simulink model "model_without_loop"  (R2022a)
settings: Solver=VariableStepAuto  StartTime=0.0  StopTime=1000  MaxStep=1e-3  RelTol=1e-3
values from neighbouring files (symbols this model uses):
  b_m = b_0    (= 7)    [config.m]
  en1 = zeros(length(Lambda), 1)    [config.m]
  gamma = 10000    [config.m]    (also in task_kras.m = 10000000000; tasks.m = 100000000; test_grad.m = 1000)
  k_0 = 1    [config.m]
  K_M = K_M_g    [config.m]
  Lambda = -k_0    (= -1)    [config.m]
  nu1 = zeros(length(Lambda), 1)    [config.m]
  nu2 = zeros(length(Lambda), 1)    [config.m]
  object_denum = [1 a_1 a_0]    [config.m]
  object_num = [b_0]    [config.m]
  psi_hat_init_conds = zeros(omega_size, 1)    [config.m]
  SysKM = ss(K_M_mat)    [config.m]
  SysMat = ss(Lmat)    [config.m]    (also in test_conf.m)
  SysVec = ss(Lvec)    [config.m]    (also in test_conf.m)
settings Model: SimulationMode=accelerator  LastModifiedBy=Vvlad
settings OptimizationCC: BlockReduction=off  BooleanDataType=off
settings DebuggingCC: SaveWithParameterizedLinksMsg=none  UnderspecifiedInitializationDetection=Classic  MergeDetectMultiDrivingBlocksExec=none  SignalResolutionControl=TryResolveAllWithWarning  UnconnectedInputMsg=warning  UnconnectedOutputMsg=warning  UnconnectedLineMsg=warning  UnderSpecifiedDimensionMsg=warning
settings HardwareCC: TargetUnknown=on
settings ModelReferenceCC: PropagateSignalLabelsOutOfModel=off
settings RTWCC: DLArmComputeVersion=19.05

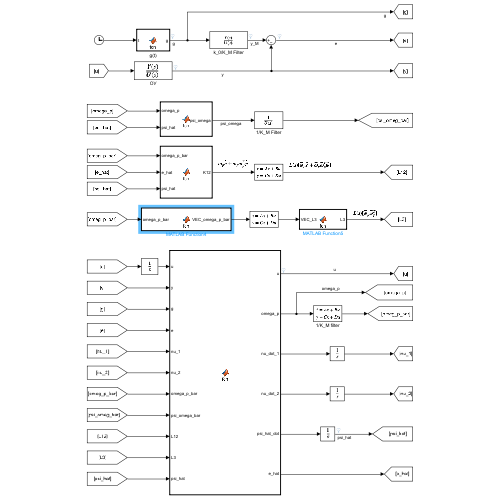
[thumbnail: Simulink's stored preview of the top-level diagram]
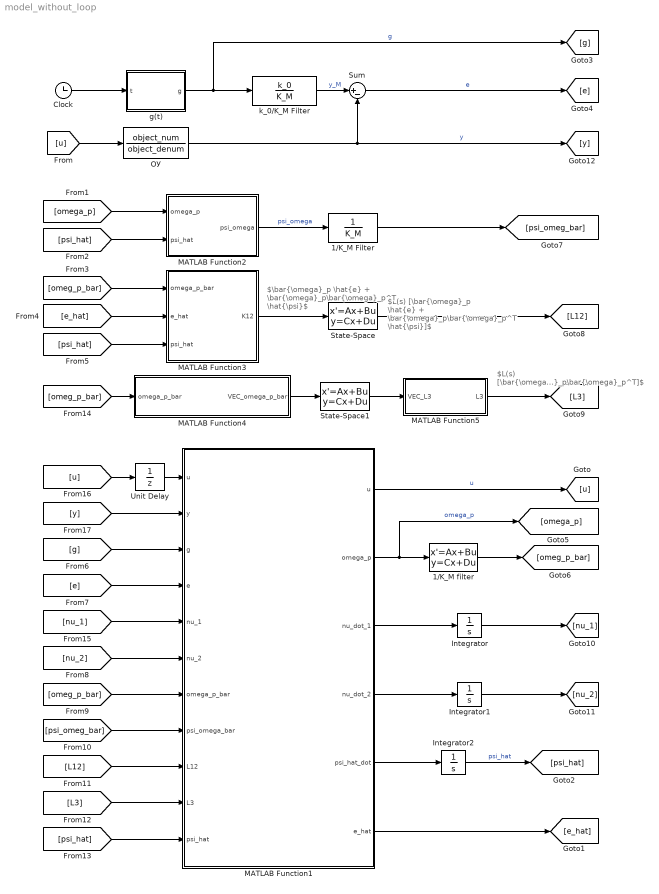
== system model_without_loop ==
  note: $L(s) [\bar{\omega}_p \hat{e} + \bar{\omega}_p\bar{\omega}_p^T \hat{\psi}]$
  note: $\bar{\omega}_p \hat{e} + \bar{\omega}_p\bar{\omega}_p^T \hat{\psi}$
  note: $L(s) [\bar{\omega}_p\bar{\omega}_p^T]$
  1/K_M Filter : TransferFcn  Denominator=K_M
  1/K_M filter : StateSpace  A=SysKM.A  B=SysKM.B  C=SysKM.C  D=SysKM.D  InitialCondition=0
  Clock : Clock
  Integrator : Integrator  InitialCondition=nu1
  Integrator1 : Integrator  InitialCondition=nu2
  Integrator2 : Integrator  InitialCondition=psi_hat_init_conds
  MATLAB Function1 : MATLAB Function  TreatAsAtomicUnit=on
  MATLAB Function2 : MATLAB Function  TreatAsAtomicUnit=on
  MATLAB Function3 : MATLAB Function  TreatAsAtomicUnit=on
  MATLAB Function4 : MATLAB Function  TreatAsAtomicUnit=on
  MATLAB Function5 : MATLAB Function  TreatAsAtomicUnit=on
  State-Space : StateSpace  A=SysVec.A  B=SysVec.B  C=SysVec.C  D=SysVec.D  InitialCondition=0
  State-Space1 : StateSpace  A=SysMat.A  B=SysMat.B  C=SysMat.C  D=SysMat.D  InitialCondition=0
  Sum : Sum  Inputs=|+-
  Unit Delay : UnitDelay  InitialCondition=[0]  SampleTime=-1  HasFrameUpgradeWarning=on
  g(t) : MATLAB Function  TreatAsAtomicUnit=on
  k_0/K_M Filter : TransferFcn  Numerator=k_0  Denominator=K_M
  ОУ : TransferFcn  Numerator=object_num  Denominator=object_denum
  wires:
  ОУ/1 -> [y], Sum/2  "y"
  Clock/1 -> g(t)/1(t)
  g(t)/1(g) -> [g], k_0/K_M Filter/1  "g"
  k_0/K_M Filter/1 -> Sum/1  "y_M"
  Sum/1 -> [e]  "e"
  [u] -> ОУ/1
  MATLAB Function1/1(u) -> [u]  "u"
  MATLAB Function3/1(K12) -> State-Space/1
  MATLAB Function1/6(e_hat) -> [e_hat]
  MATLAB Function1/5(psi_hat_dot) -> Integrator2/1
  Integrator2/1 -> [psi_hat]  "psi_hat"
  1/K_M Filter/1 -> [psi_omeg_bar]
  MATLAB Function2/1(psi_omega) -> 1/K_M Filter/1  "psi_omega"
  [omega_p] -> MATLAB Function2/1(omega_p)
  [psi_hat] -> MATLAB Function2/2(psi_hat)
  [psi_hat] -> MATLAB Function3/3(psi_hat)
  [e_hat] -> MATLAB Function3/2(e_hat)
  [omeg_p_bar] -> MATLAB Function3/1(omega_p_bar)
  State-Space/1 -> [L12]
  [g] -> MATLAB Function1/3(g)
  [omeg_p_bar] -> MATLAB Function1/7(omega_p_bar)
  [psi_omeg_bar] -> MATLAB Function1/8(psi_omega_bar)
  [L12] -> MATLAB Function1/9(L12)
  [L3] -> MATLAB Function1/10(L3)
  [psi_hat] -> MATLAB Function1/11(psi_hat)
  State-Space1/1 -> MATLAB Function5/1(VEC_L3)
  [omeg_p_bar] -> MATLAB Function4/1(omega_p_bar)
  MATLAB Function4/1(VEC_omega_p_bar) -> State-Space1/1
  MATLAB Function5/1(L3) -> [L3]
  1/K_M filter/1 -> [omeg_p_bar]
  MATLAB Function1/2(omega_p) -> 1/K_M filter/1, [omega_p]  "omega_p"
  MATLAB Function1/4(nu_dot_2) -> Integrator1/1
  MATLAB Function1/3(nu_dot_1) -> Integrator/1
  Integrator/1 -> [nu_1]
  Integrator1/1 -> [nu_2]
  [nu_2] -> MATLAB Function1/6(nu_2)
  [nu_1] -> MATLAB Function1/5(nu_1)
  [e] -> MATLAB Function1/4(e)
  [y] -> MATLAB Function1/2(y)
  [u] -> Unit Delay/1
  Unit Delay/1 -> MATLAB Function1/1("u ")

== matlab function model_without_loop/g(t) ==
  data: t input; g output
function g = fcn(t)

g = 7*sin(8*t+1);

== matlab function model_without_loop/MATLAB Function1 ==
  data: u input; u output size=1; y input; g input; e input; nu_1 input; nu_2 input; omega_p output; nu_dot_1 output; nu_dot_2 output; omega_p_bar input; psi_hat_dot output; psi_omega_bar input; L12 input; L3 input; psi_hat input; gamma parameter; k_0 parameter; b_m parameter; e_hat output double; Lambda parameter; en1 parameter
function [u, omega_p, nu_dot_1, nu_dot_2, psi_hat_dot, e_hat] = fcn(u, y, g, e, nu_1, nu_2, omega_p_bar, psi_omega_bar, L12, L3, psi_hat, gamma, k_0, b_m, Lambda, en1)

nu_dot_1 = Lambda*nu_1 + en1*u;
nu_dot_2 = Lambda*nu_2 + en1*y;
omega = [nu_1', nu_2', y]';
omega_p = -omega;

% psi_hat = [-31.3957;2.8152; 44.7236];
e_hat = e - psi_hat'*omega_p_bar + psi_omega_bar;
psi_hat_dot = gamma*(L12 - L3*psi_hat);
u = (psi_hat'*omega_p+k_0*g)/b_m;

== matlab function model_without_loop/MATLAB Function2 ==
  data: omega_p input; psi_hat input; psi_omega output
function psi_omega = fcn(omega_p, psi_hat)
psi_omega = psi_hat'*omega_p;

== matlab function model_without_loop/MATLAB Function3 ==
  data: omega_p_bar input; K12 output; e_hat input; psi_hat input
function K12 = fcn(omega_p_bar, e_hat, psi_hat)

K12 = omega_p_bar*e_hat + omega_p_bar*omega_p_bar'*psi_hat;

== matlab function model_without_loop/MATLAB Function4 ==
  data: omega_p_bar input; VEC_omega_p_bar output
function VEC_omega_p_bar = fcn(omega_p_bar)

VEC_omega_p_bar = reshape(omega_p_bar*omega_p_bar', length(omega_p_bar)^2, 1);

== matlab function model_without_loop/MATLAB Function5 ==
  data: VEC_L3 input; L3 output
function L3 = fcn(VEC_L3)
L3 = reshape(VEC_L3, sqrt(length(VEC_L3)), sqrt(length(VEC_L3)));
